simulink model "PendulumRobotArm_CloseLoop"  (R2019a)
settings: Solver=VariableStepAuto  StartTime=0.0  StopTime=20  RelTol=1e-3
values from neighbouring files (symbols this model uses):
  c = 1.0791e-5    (= 1.0791e-05)    [Parameters.m]
  g = 9.81    [Parameters.m]
  J = J_motor + m*l^2 + I    (= 0.0704425)    [Parameters.m]
  ke = 50.68*60/(2*pi*1000)    (= 0.483958350954)    [Parameters.m]
  km = 0.415    [Parameters.m]
  l = 3/8    (= 0.375)    [Parameters.m]
  L = 4.8*1e-3    (= 0.0048)    [Parameters.m]
  m = 1/4    (= 0.25)    [Parameters.m]
  R = 9.65    [Parameters.m]
libraries: simulink x1
settings Model: Creator=sp_ja  LastModifiedBy=sp_ja

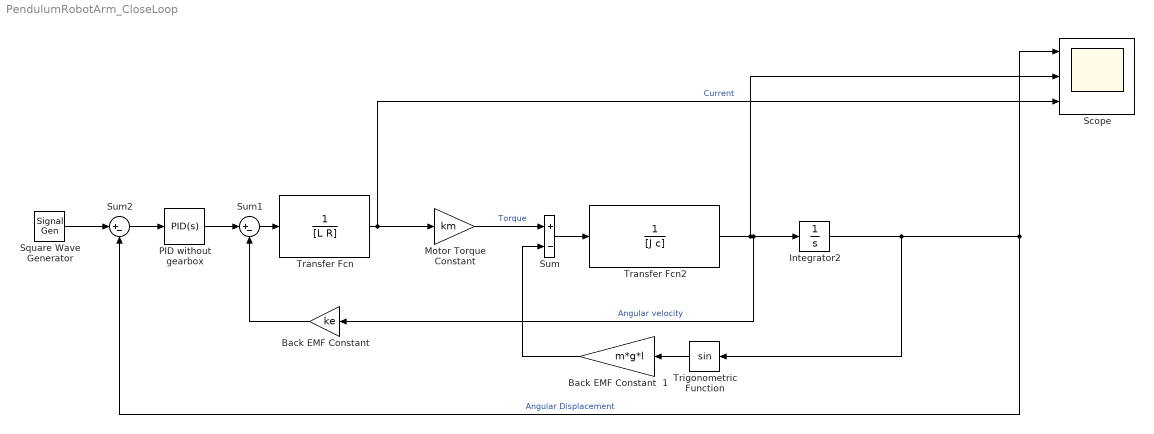
== system PendulumRobotArm_CloseLoop ==
  "Back EMF Constant  " : Gain  Gain=ke
  Back EMF Constant  1 : Gain  Gain=m*g*l
  "Integrator2 " : Integrator  InitialCondition=0*pi/180
  Motor Torque Constant : Gain  Gain=km
  PID without gearbox : simulink/Continuous/PID Controller  Controller=PID  Form=Parallel  TimeDomain=Continuous-time  SampleTime=-1  IntegratorMethod=Forward Euler  FilterMethod=Forward Euler  ControllerParametersSource=internal  P=60.47435050807  I=57.6366194816351  D=9.55264495495961  UseFilter=on  N=12.9132594842849  TunerSelectOption=Transfer Function Based (PID Tuner App)  InitialConditionSource=internal  InitialConditionForIntegrator=0  InitialConditionForFilter=0  DifferentiatorICPrevScaledInput=0  ExternalReset=none  TrackingMode=off  Kt=1  LimitOutput=off  UpperSaturationLimit=inf  LowerSaturationLimit=-inf  LinearizeAsGain=on  AntiWindupMode=none  Kb=1  POutMin=[]  POutMax=[]  IOutMin=[]  IOutMax=[]  DOutMin=[]  DOutMax=[]  NOutMin=[]  NOutMax=[]  SumOutMin=[]  SumOutMax=[]  SaturationOutMin=[]  SaturationOutMax=[]  PParamMin=[]  PParamMax=[]  IParamMin=[]  IParamMax=[]  DParamMin=[]  DParamMax=[]  NParamMin=[]  NParamMax=[]  KbParamMin=[]  KbParamMax=[]  KtParamMin=[]  KtParamMax=[]  KbOutMin=[]  KbOutMax=[]  KtOutMin=[]  KtOutMax=[]  IntegratorOutMin=[]  IntegratorOutMax=[]  FilterOutMin=[]  FilterOutMax=[]  SumI1OutMin=[]  SumI1OutMax=[]  SumI2OutMin=[]  SumI2OutMax=[]  SumI3OutMin=[]  SumI3OutMax=[]  SumI4OutMin=[]  SumI4OutMax=[]  SumDOutMin=[]  SumDOutMax=[]  DifferentiatorOutMin=[]  DifferentiatorOutMax=[]  FilterDiffOutCoefMin=[]  FilterDiffOutCoefMax=[]  ReciprocalOutMin=[]  ReciprocalOutMax=[]  SumDenOutMin=[]  SumDenOutMax=[]  SumNumOutMin=[]  SumNumOutMax=[]  DivideOutMin=[]  DivideOutMax=[]  IntegratorContinuousStateAttributes=''  IntegratorStateMustResolveToSignalObject=off  IntegratorRTWStateStorageClass=Auto  FilterContinuousStateAttributes=''  FilterStateMustResolveToSignalObject=off  FilterRTWStateStorageClass=Auto  ParallelPVariant=InternalParameters  IdealPVariant=Disabled  IVariant=InternalParameters  DVariant=InternalParameters  IntegratorVariant=Continuous  SatVariant=Disabled  AWVariant=Passthrough  PCopyVariant=Disabled  TRVariant=Disabled  FdbkBlocksVariant=Forward  IdealPFdbkVariant=Disabled  SatFdbkVariant=Disabled  DerivativeFilterVariant=ContFilter  NVariant=InternalParameters  NCopyVariant=Disabled  FilterICVariant=InternalICsFilter  IntegratorICVariant=InternalICs  ExternalResetVariant=Disabled  TRSumVariant=Passthrough  SumFdbkVariant=Disabled  SumVariant=Sum_PID
  "Scope " : Scope  NumInputPorts=3
  "Square Wave Generator " : SignalGenerator  WaveForm=square  Frequency=0.1
  Sum : Sum  Inputs=+-
  Sum1 : Sum  Inputs=|+-
  Sum2 : Sum  Inputs=|+-
  "Transfer Fcn " : TransferFcn  Denominator=[L R]
  "Transfer Fcn2 " : TransferFcn  Denominator=[J c]
  Trigonometric Function : Trigonometry
  wires:
  Sum/1 -> "Transfer Fcn2 "/1
  Sum1/1 -> "Transfer Fcn "/1
  "Back EMF Constant  "/1 -> Sum1/2
  "Transfer Fcn "/1 -> Motor Torque Constant/1, "Scope "/3  "Current"
  "Integrator2 "/1 -> Trigonometric Function/1, Sum2/2, "Scope "/1  "Angular Displacement"
  PID without gearbox/1 -> Sum1/1
  Sum2/1 -> PID without gearbox/1
  "Square Wave Generator "/1 -> Sum2/1
  Motor Torque Constant/1 -> Sum/1  "Torque"
  "Transfer Fcn2 "/1 -> "Back EMF Constant  "/1, "Integrator2 "/1, "Scope "/2  "Angular velocity"
  Trigonometric Function/1 -> Back EMF Constant  1/1
  Back EMF Constant  1/1 -> Sum/2
